simulink model "Puissance"  (R2024b)
settings: Solver=VariableStepAuto  StartTime=0.0  StopTime=0.02  MaxStep=1e-3  RelTol=1e-3
values from neighbouring files (symbols this model uses):
  Te = 1e-3    (= 0.001)    [defvars.m]
  Tf = 0.2    [defvars.m]
undefined symbols (not defined in the file or in its folder): DiscIntNeverNeededParam
libraries: simulink x2
settings Model: Creator=marc.nicoller  LastModifiedBy=marc.nicoller

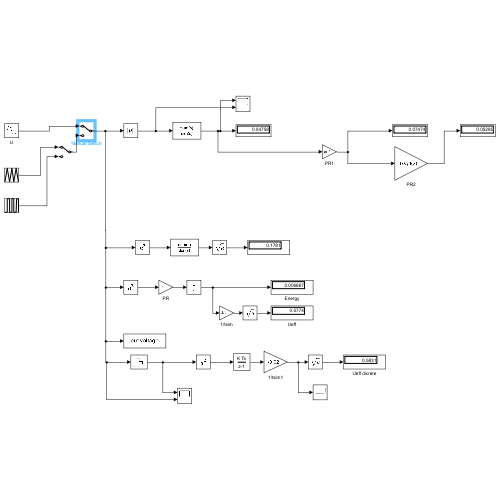
[thumbnail: Simulink's stored preview of the top-level diagram]
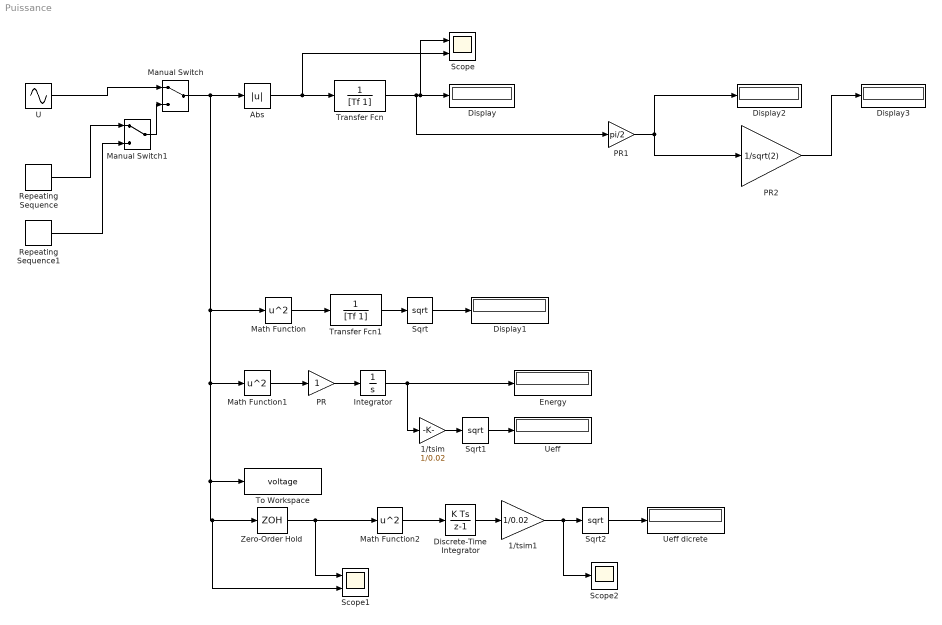
== system Puissance ==
  1/tsim : Gain  Gain=1/0.02
  1/tsim1 : Gain  Gain=1/0.02
  Abs : Abs  SaturateOnIntegerOverflow=off
  Discrete-Time Integrator : DiscreteIntegrator  SampleTime=Te  ICPrevOutput=DiscIntNeverNeededParam  ICPrevScaledInput=DiscIntNeverNeededParam
  Display{,1..3} (4 alike) : Display
  Energy : Display
  Integrator : Integrator
  Manual Switch : ManualSwitch
  Manual Switch1 : ManualSwitch
  Math Function : Math  Operator=square
  Math Function1 : Math  Operator=square
  Math Function2 : Math  Operator=square
  PR : Gain
  PR1 : Gain  Gain=pi/2
  PR2 : Gain  Gain=1/sqrt(2)
  Repeating Sequence : simulink/Sources/Repeating Sequence  rep_seq_t=[0 0.01 0.02]  rep_seq_y=[-1 1 -1]
  Repeating Sequence1 : simulink/Sources/Repeating Sequence  rep_seq_t=[0 0.01 0.011 0.02]  rep_seq_y=[-1 -1 1 1]
  Scope : Scope  NumInputPorts=2
  Scope1 : Scope  NumInputPorts=2
  Scope2 : Scope
  Sqrt : Sqrt
  Sqrt1 : Sqrt
  Sqrt2 : Sqrt
  To Workspace : ToWorkspace  VariableName=voltage  SaveFormat=Timeseries  SampleTime=Te
  Transfer Fcn : TransferFcn  Denominator=[Tf 1]
  Transfer Fcn1 : TransferFcn  Denominator=[Tf 1]
  U : Sin  Frequency=2*pi*50  SampleTime=0
  Ueff : Display
  Ueff dicrete : Display
  Zero-Order Hold : ZeroOrderHold  SampleTime=Te
  wires:
  Manual Switch/1 -> Scope1/2, Zero-Order Hold/1, To Workspace/1, Math Function1/1, Math Function/1, Abs/1
  Abs/1 -> Scope/2, Transfer Fcn/1
  Transfer Fcn/1 -> PR1/1, Scope/1, Display/1
  Math Function/1 -> Transfer Fcn1/1
  Transfer Fcn1/1 -> Sqrt/1
  Sqrt/1 -> Display1/1
  U/1 -> Manual Switch/1
  Repeating Sequence/1 -> Manual Switch1/1
  Math Function1/1 -> PR/1
  PR/1 -> Integrator/1
  Integrator/1 -> Energy/1, 1/tsim/1
  Sqrt1/1 -> Ueff/1
  1/tsim/1 -> Sqrt1/1
  Manual Switch1/1 -> Manual Switch/2
  Repeating Sequence1/1 -> Manual Switch1/2
  Zero-Order Hold/1 -> Math Function2/1, Scope1/1
  Math Function2/1 -> Discrete-Time Integrator/1
  Sqrt2/1 -> Ueff dicrete/1
  Discrete-Time Integrator/1 -> 1/tsim1/1
  1/tsim1/1 -> Scope2/1, Sqrt2/1
  PR1/1 -> Display2/1, PR2/1
  PR2/1 -> Display3/1
